simulink model "Pump_Series"  (R2018b)
settings: Solver=VariableStepAuto  StartTime=0.0  StopTime=200  MaxStep=1  RelTol=1e-3  EnableMultiTasking=on
undefined symbols (not defined in the file): path_carnot
libraries: carnot x5, simulink x2
settings Model: Creator=drhf  LastModifiedBy=drhf
settings DataIOCC: LimitDataPoints=on  SaveFormat=Array  SignalLoggingSaveFormat=ModelDataLogs
settings OptimizationCC: ExpressionDepthLimit=2147483647  LifeSpan=inf
settings DebuggingCC: UnderspecifiedInitializationDetection=Classic  MergeDetectMultiDrivingBlocksExec=none  SolverPrmCheckMsg=warning  StateNameClashWarn=warning  SFUnexpectedBacktrackingDiag=warning  SFNoUnconditionalDefaultTransitionDiag=warning  SFExecutionAtInitializationDiag=none
settings HardwareCC: ProdBitPerPointer=32  ProdBitPerSizeT=32  ProdBitPerPtrDiffT=32  ProdLargestAtomicFloat=None  ProdIntDivRoundTo=Undefined  ProdEndianess=Unspecified  ProdWordSize=32  ProdHWDeviceType=32-bit Generic
settings ModelReferenceCC: PropagateSignalLabelsOutOfModel=off
settings SFSimCC: SimUseLocalCustomCode=off
settings RTWCC: RTWUseLocalCustomCode=off
settings CodeAppCC: StateflowObjectComments=on
settings GRTTargetCC: TargetLangStandard=C89/C90 (ANSI)  GeneratePreprocessorConditionals=Disable all  CombineOutputUpdateFcns=off  GRTInterface=on
settings ConfigComp: CovMetricSettings=dw  CovHtmlReporting=on  CovSaveCumulativeToWorkspaceVar=on  CovSaveSingleToWorkspaceVar=on  CovExternalEMLEnable=off

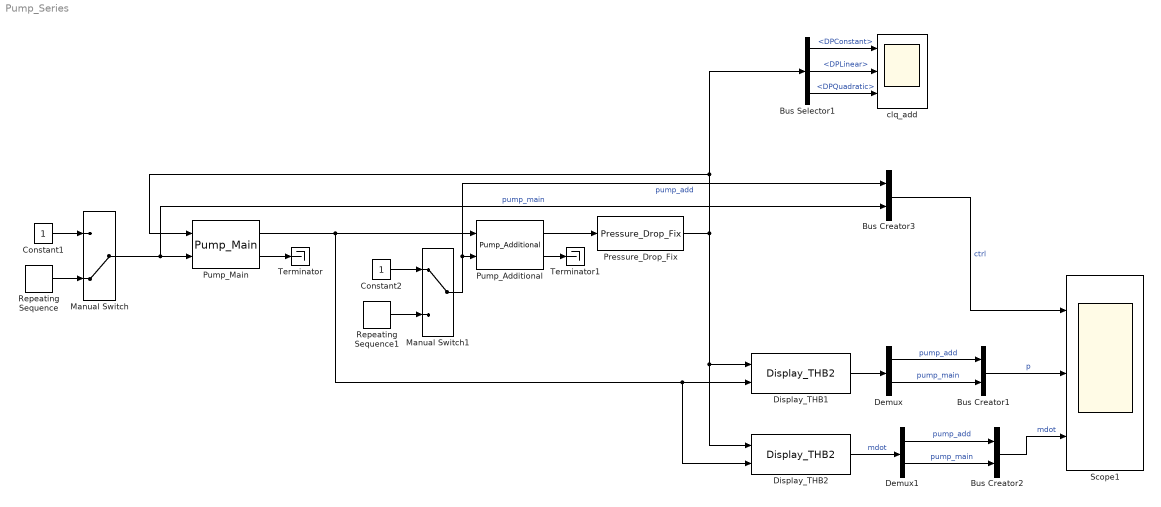
== system Pump_Series ==
  Bus Creator1 : BusCreator  Inputs=2
  Bus Creator2 : BusCreator  Inputs=2
  Bus Creator3 : BusCreator  Inputs=2
  Bus Selector1 : BusSelector  OutputSignals=DPConstant,DPLinear,DPQuadratic
  Constant1 : Constant
  Constant2 : Constant
  Demux : Demux  Outputs=2
  Demux1 : Demux  Outputs=2
  Display_THB1 : carnot/Outputs/Display_THB2  t=off  m=off  p=on  id=off  mix=off  d=off
  Display_THB2 : carnot/Outputs/Display_THB2  t=off  m=on  p=off  id=off  mix=off  d=off
  Manual Switch : ManualSwitch  CurrentSetting=0
  Manual Switch1 : ManualSwitch
  Pressure_Drop_Fix : carnot/Basic/Pressure_Drop/Pressure_Drop_Fix  con=0  lin=0  qua=0
  Pump_Additional : carnot/Hydraulics/Pump_Additional  Tini=20  PathName=fullfile(path_carnot('libsl'), 'Hydraulics', 'Pump_Main', 'parameter_set')  FileName='Pump6m.mat'  userPath=off  userParam=off  a0=60000  a1=-43200  a2=0  dia=0.025  UA=1  mcp=4182  e0=50  e1=28.8  e2=-10.368
  Pump_Main : carnot/Hydraulics/Pump_Main  Tini=20  p0=3e5  IDpreset=pressure drop  fluid=Water  mix=0  mix2=0  mix3=0  t1=1  PathName=fullfile(path_carnot('libsl'), 'Hydraulics', 'Pump_Main', 'parameter_set')  FileName='Pump6m.mat'  userPath=off  userParam=off  a0=60000  a1=-43200  a2=0  dia=0.025  UA=1  mcp=4182  e0=50  e1=28.8  e2=-10.368
  Repeating Sequence : simulink/Sources/Repeating Sequence  rep_seq_t=[0 20 60 120 180 200]  rep_seq_y=[0 0 1 1 0 0]
  Repeating Sequence1 : simulink/Sources/Repeating Sequence  rep_seq_t=[0 20 60 120 180 200]  rep_seq_y=[0 0 1 1 0 0]
  Scope1 : Scope  NumInputPorts=3
  Terminator : Terminator
  Terminator1 : Terminator
  clq_add : Scope  NumInputPorts=3
  wires:
  Pump_Main/2 -> Terminator/1
  Pressure_Drop_Fix/1 -> Display_THB2/1, Display_THB1/1, Pump_Main/1, Bus Selector1/1
  Display_THB1/1 -> Demux/1
  Demux/1 -> Bus Creator1/1  "pump_add"
  Demux/2 -> Bus Creator1/2  "pump_main"
  Bus Creator1/1 -> Scope1/2  "p"
  Repeating Sequence/1 -> Manual Switch/2
  Constant1/1 -> Manual Switch/1
  Bus Creator2/1 -> Scope1/3  "mdot"
  Demux1/1 -> Bus Creator2/1  "pump_add"
  Demux1/2 -> Bus Creator2/2  "pump_main"
  Display_THB2/1 -> Demux1/1  "mdot"
  Pump_Main/1 -> Pump_Additional/1, Display_THB2/2, Display_THB1/2
  Pump_Additional/1 -> Pressure_Drop_Fix/1
  Pump_Additional/2 -> Terminator1/1
  Constant2/1 -> Manual Switch1/1
  Repeating Sequence1/1 -> Manual Switch1/2
  Bus Selector1/3 -> clq_add/3  "<DPQuadratic>"
  Bus Selector1/1 -> clq_add/1  "<DPConstant>"
  Bus Selector1/2 -> clq_add/2  "<DPLinear>"
  Manual Switch/1 -> Bus Creator3/2, Pump_Main/2  "pump_main"
  Manual Switch1/1 -> Bus Creator3/1, Pump_Additional/2  "pump_add"
  Bus Creator3/1 -> Scope1/1  "ctrl"
